simulink model "sim_ES01_02"  (R2021b)
settings: Solver=VariableStepAuto  StartTime=0.0  StopTime=10.0  MaxStep=1e-02  RelTol=1e-3
values from neighbouring files (symbols this model uses):
  c = 2664    [DatiSospensione.m]    (also in Dati_Necessari.m; ES01_Comfort_4dof_stud.m = 0.00047; ES2_2DOF.m = C_values(count2); ES_2DOF_ANIM_TF.m = c_opt)
  h0 = 2/100    (= 0.02)    [Dati_Necessari.m]    (also in ES01_Comfort_4dof_stud.m = 0.01; ES_2DOF_ANIM_TF.m)
  k = 35495    [DatiSospensione.m]    (also in Dati_Necessari.m = 99000; ES2_2DOF.m = 99000)
  lambda = 2    [Dati_Necessari.m]    (also in ES01_Comfort_4dof_stud.m = 2*pi*V./OM; ES_2DOF_ANIM_TF.m)
  m = ms+mu    (= 395)    [DatiSospensione.m]    (also in ES01_Comfort_4dof_stud.m = 1790)
  v = 0    [Dati_Necessari.m]    (also in ES_2DOF_ANIM_TF.m = 36.1111111111)
  z0 = 0    [Dati_Necessari.m]    (also in ES_2DOF_ANIM_TF.m)
  zd0 = 0    [Dati_Necessari.m]    (also in ES_2DOF_ANIM_TF.m)
settings Model: Creator=Utente  LastModifiedBy=Utente
settings DataIOCC: ReturnWorkspaceOutputs=off

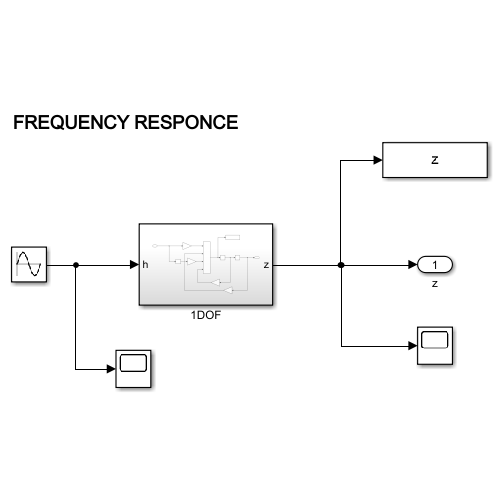
[thumbnail: Simulink's stored preview of the top-level diagram]
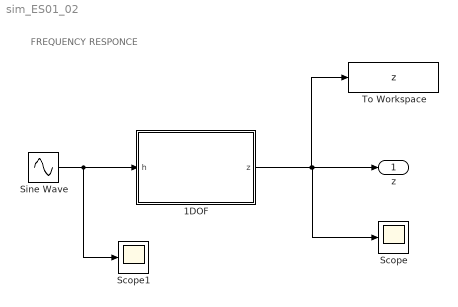
== system sim_ES01_02 ==
  note: FREQUENCY RESPONCE
  1DOF : Subsystem
  Scope : Scope
  Scope1 : Scope
  Sine Wave : Sin  Amplitude=h0  Frequency=2*pi*v/lambda  SampleTime=0
  To Workspace : ToWorkspace  VariableName=z  SaveFormat=Timeseries  SampleTime=-1
  z : Outport
  wires:
  1DOF/1(z) -> To Workspace/1, Scope/1, z/1
  Sine Wave/1 -> Scope1/1, 1DOF/1(h)

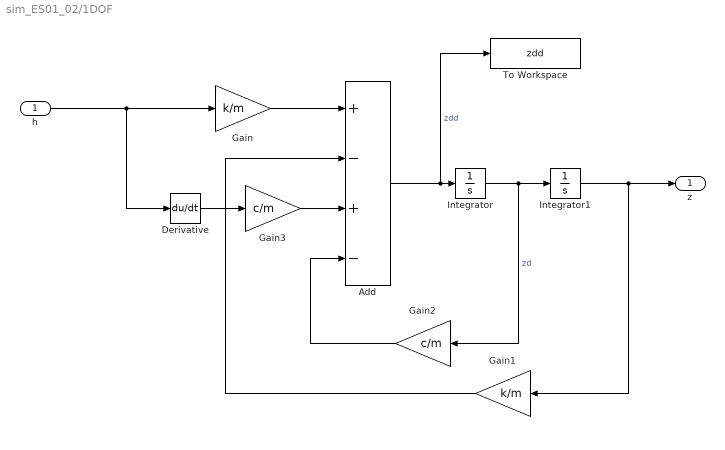
== system sim_ES01_02/1DOF ==
  h : Inport
  Add : Sum  Inputs=+-+-
  Derivative : Derivative
  Gain : Gain  Gain=k/m
  Gain1 : Gain  Gain=k/m
  Gain2 : Gain  Gain=c/m
  Gain3 : Gain  Gain=c/m
  Integrator : Integrator  InitialCondition=zd0
  Integrator1 : Integrator  InitialCondition=z0
  To Workspace : ToWorkspace  VariableName=zdd  SaveFormat=Timeseries  SampleTime=-1
  z : Outport
  wires:
  Derivative/1 -> Gain3/1
  Add/1 -> To Workspace/1, Integrator/1  "zdd"
  h/1 -> Derivative/1, Gain/1
  Gain1/1 -> Add/2
  Integrator1/1 -> z/1, Gain1/1
  Gain/1 -> Add/1
  Gain3/1 -> Add/3
  Integrator/1 -> Gain2/1, Integrator1/1  "zd"
  Gain2/1 -> Add/4
